simulink model "rawmotor_sim"  (Simulink 8.8)
settings: Solver=FixedStepDiscrete  StartTime=0.0  StopTime=10.0  RelTol=1e-3
libraries: sphero_lib x4
settings Model: Creator=gcampa  LastModifiedBy=gcampa
settings DataIOCC: SignalLoggingSaveFormat=Dataset
settings OptimizationCC: BlockReduction=off  BooleanDataType=off
settings DebuggingCC: SaveWithParameterizedLinksMsg=none  SignalResolutionControl=TryResolveAllWithWarning  FcnCallInpInsideContextMsg=error  StateNameClashWarn=none
settings HardwareCC: TargetUnknown=on
settings GRTTargetCC: CombineOutputUpdateFcns=on  GRTInterface=off

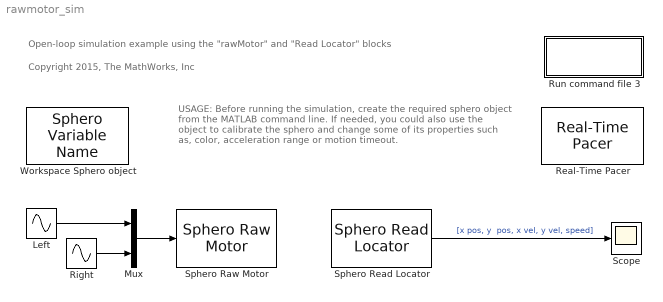
== system rawmotor_sim ==
  note: Copyright 2015, The MathWorks, Inc
  note: USAGE:
      | Before running the simulation, create the required sphero object
      | from the MATLAB command line. If needed, you could also use
      | the object to calibrate the sphero and change some of its properties
      | such as, color, acceleration range or motion timeout.
  note: Open-loop simulation example using the "rawMotor" and "Read Locator" blocks
  Left : Sin  Amplitude=100  Frequency=pi/2/5  SampleTime=1
  Mux : Mux  Inputs=[1 1]
  Real-Time Pacer : sphero_lib/Real-Time Pacer  simTimePerRealTime=1
  Right : Sin  Amplitude=100  Frequency=pi/2/5  Phase=pi/2  SampleTime=1
  Run command file 3 : Subsystem
      settings: OpenFcn=sphero_lib
      mask Display: disp('Open Main\nSimulink Library')
  Scope : Scope
  Sphero Raw Motor : sphero_lib/Sphero Raw Motor  SpheroVarNumber=Existing workspace Sphero variable #1  T=0.2
  Sphero Read Locator : sphero_lib/Sphero Read Locator  SpheroVarNumber=Existing workspace Sphero variable #1  T=0.2
  Workspace Sphero object : sphero_lib/Sphero Variable Name  Priority=3  SpheroVarNumber=Existing workspace Sphero variable #1  workspaceVarName=sph
  wires:
  Sphero Read Locator/1 -> Scope/1  "[x pos, y  pos, x vel, y vel, speed]"
  Right/1 -> Mux/2
  Left/1 -> Mux/1
  Mux/1 -> Sphero Raw Motor/1

== system rawmotor_sim/Run command file 3 ==
